simulink model "untitled"  (R2022a)
settings: Solver=ode5  StartTime=0.0  StopTime=10.0  FixedStep=0.1  RelTol=1e-3  EnableMultiTasking=on
settings Model: Creator=luiz_  LastModifiedBy=lucas
settings SolverCC: AlgebraicLoopSolver=TrustRegion
settings DataIOCC: ReturnWorkspaceOutputs=off
settings OptimizationCC: LifeSpan=inf
settings DebuggingCC: UnconnectedInputMsg=warning  UnconnectedOutputMsg=warning  UnconnectedLineMsg=warning  SFUnexpectedBacktrackingDiag=warning  SFNoUnconditionalDefaultTransitionDiag=warning  SFMachineParentedDataDiag=warning  ArithmeticOperatorsInVariantConditions=warning
settings SFSimCC: SimUseLocalCustomCode=off  CustomCodeUndefinedFunction=UseInterfaceOnly
settings RTWCC: RTWUseLocalCustomCode=off
settings CodeAppCC: StateflowObjectComments=on
settings GRTTargetCC: TargetLangStandard=C89/C90 (ANSI)
settings ConfigComp: CovMetricSettings=dw  CovSaveCumulativeToWorkspaceVar=on  CovSaveSingleToWorkspaceVar=on  CovExternalEMLEnable=off

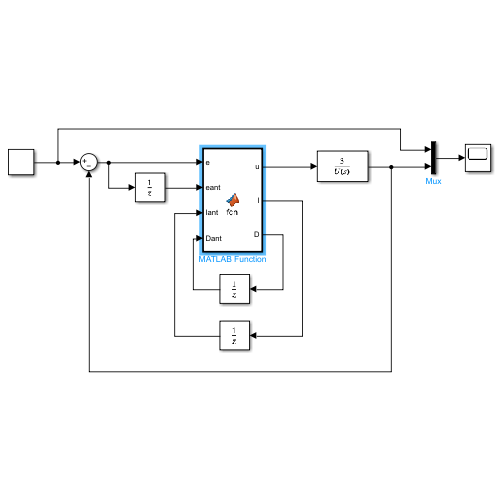
[thumbnail: Simulink's stored preview of the top-level diagram]
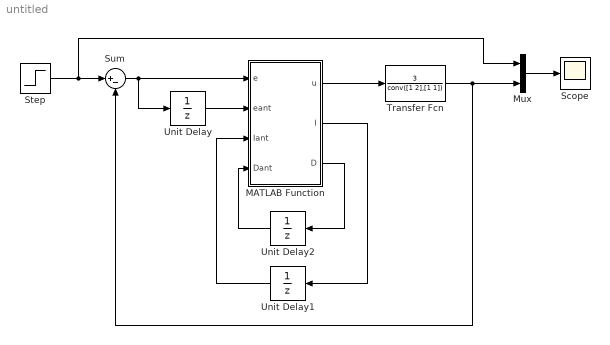
== system untitled ==
  MATLAB Function : MATLAB Function  TreatAsAtomicUnit=on
  Mux : Mux  Inputs=2
  Scope : Scope
  Step : Step  Time=0  After=2  SampleTime=0
  Sum : Sum  Inputs=|+-
  Transfer Fcn : TransferFcn  Numerator=[3]  Denominator=conv([1 2],[1 1])
  Unit Delay : UnitDelay  SampleTime=0.1  HasFrameUpgradeWarning=on
  Unit Delay1 : UnitDelay  SampleTime=0.1  HasFrameUpgradeWarning=on
  Unit Delay2 : UnitDelay  SampleTime=0.1  HasFrameUpgradeWarning=on
  wires:
  MATLAB Function/1(u) -> Transfer Fcn/1
  Transfer Fcn/1 -> Mux/2, Sum/2
  Step/1 -> Mux/1, Sum/1
  Sum/1 -> Unit Delay/1, MATLAB Function/1(e)
  Unit Delay/1 -> MATLAB Function/2(eant)
  MATLAB Function/2(I) -> Unit Delay1/1
  Unit Delay1/1 -> MATLAB Function/3(Iant)
  MATLAB Function/3(D) -> Unit Delay2/1
  Unit Delay2/1 -> MATLAB Function/4(Dant)
  Mux/1 -> Scope/1

== matlab function untitled/MATLAB Function ==
  data: e input; eant input; u output; Iant input; I output; Dant input; D output
function [u,I,D] = fcn(e,eant, Iant, Dant)

T = 0.1;
Kp = 2.534;
Kd = 0.6/Kp;
Ki = 2.668/Kp;

P = Kp*e;
I = (Iant + ((Ki*T)/2)*(e + eant));
D = (-Dant + ((2*Kd)/T)*(e - eant));



u=P+I+D;
